simulink model "rest_vector_data_task"  (Simulink 3.00)
libraries: mathlib x5, matrixlib x1, arclib x1

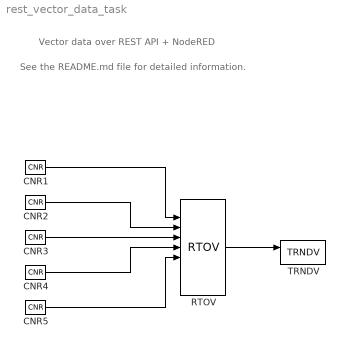
== system rest_vector_data_task ==
  note: See the README.md file for detailed information.
  note: Vector data over REST API + NodeRED
  CNR1 : mathlib/CNR  ycn=3.0
  CNR2 : mathlib/CNR  ycn=5.7
  CNR3 : mathlib/CNR  ycn=6.5
  CNR4 : mathlib/CNR  ycn=7.8
  CNR5 : mathlib/CNR  ycn=12
  RTOV : matrixlib/RTOV  nmax=5  offset=0  n=5  etype=8: Double
  TRNDV : arclib/TRNDV  n=5  l=2  btype=8: Double  pfac=1  afac=0  arc=0  id=1  Title=Trend Title  timesrc=1: CORETIMER
  wires:
  CNR1/1 -> RTOV/2
  CNR2/1 -> RTOV/3
  CNR3/1 -> RTOV/4
  CNR4/1 -> RTOV/5
  CNR5/1 -> RTOV/6
  RTOV/1 -> TRNDV/1
